simulink model "TransitionCommonEvent_2018a"  (R2018a)
settings: Solver=VariableStepAuto  StartTime=0.0  StopTime=10.0  RelTol=1e-3
settings Model: Creator=apple  LastModifiedBy=apple
settings DataIOCC: ReturnWorkspaceOutputs=on
settings SFSimCC: SimUseLocalCustomCode=on
settings RTWCC: RTWUseLocalCustomCode=on

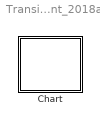
== system TransitionCommonEvent_2018a ==
  Chart : Stateflow chart  TreatAsAtomicUnit=on

== stateflow chart TransitionCommonEvent_2018a/Chart ==
  state A
    en:fprintf("Entry A");
    du:fprintf("During A");
    ex:fprintf("Exit A");
  state C
    en:fprintf("Entry C");
    du:fprintf("During C");
    ex:fprintf("Exit A");
  state B
    en:fprintf("Entry B");
    du:fprintf("During B");
    ex:fprintf("Exit B");
  (default) -> A
  A -> (junction 8) [order 2]
  (junction 8) -> C : E_one
  A -> B [order 1] : E_one
  B -> (junction 8)
  events: E_one local FUNCTION_CALL_EVENT
